simulink model "kalman"  (R2020b)
settings: Solver=VariableStepAuto  StartTime=0.0  StopTime=60  RelTol=1e-3
values from neighbouring files (symbols this model uses):
  dt_sample = 0.01    [main.m]
  dt_sensor = 5    [main.m]
  dt_sim = 0.001    [main.m]
  J = 0.7    [main.m]
  P0 = diag([(10*pi/180)^2;(1*pi/180)^2])    [main.m]
  seedv = randi(2^32)    [main.m]
  seedw = randi(2^32)    [main.m]
  sigmav = 1*pi/180    (= 0.0174532925199)    [main.m]
  sigmaw = 0.001    [main.m]
  x0_hat = [0;0]    [main.m]
libraries: simulink x1
settings Model: Creator=tjones  LastModifiedBy=tjones

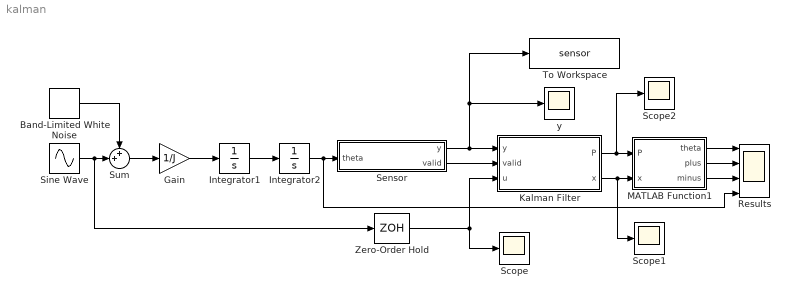
== system kalman ==
  Band-Limited White Noise : simulink/Sources/Band-Limited White Noise  Cov=[sigmaw^2]  Ts=dt_sim  seed=[seedw]
  Gain : Gain  Gain=1/J
  Integrator1 : Integrator
  Integrator2 : Integrator
  Kalman Filter : Subsystem
  MATLAB Function1 : MATLAB Function  TreatAsAtomicUnit=on
  Results : Scope  NumInputPorts=4
  Scope : Scope
  Scope1 : Scope
  Scope2 : Scope
  Sensor : Subsystem
  Sine Wave : Sin  Amplitude=0  SampleTime=dt_sim
  Sum : Sum  Inputs=++|
  To Workspace : ToWorkspace  VariableName=sensor  SaveFormat=Timeseries  SampleTime=-1
  Zero-Order Hold : ZeroOrderHold  SampleTime=dt_sample
  y : Scope
  wires:
  Integrator1/1 -> Integrator2/1
  Integrator2/1 -> Results/4, Sensor/1(theta)
  Sensor/1(y) -> Kalman Filter/1(y), y/1, To Workspace/1
  Gain/1 -> Integrator1/1
  Sine Wave/1 -> Sum/2, Zero-Order Hold/1
  Sum/1 -> Gain/1
  Zero-Order Hold/1 -> Scope/1, Kalman Filter/3(u)
  Sensor/2(valid) -> Kalman Filter/2(valid)
  Kalman Filter/1(P) -> Scope2/1, MATLAB Function1/1(P)
  Kalman Filter/2(x) -> Scope1/1, MATLAB Function1/2(x)
  MATLAB Function1/1(theta) -> Results/1
  MATLAB Function1/2(plus) -> Results/2
  MATLAB Function1/3(minus) -> Results/3
  Band-Limited White Noise/1 -> Sum/1

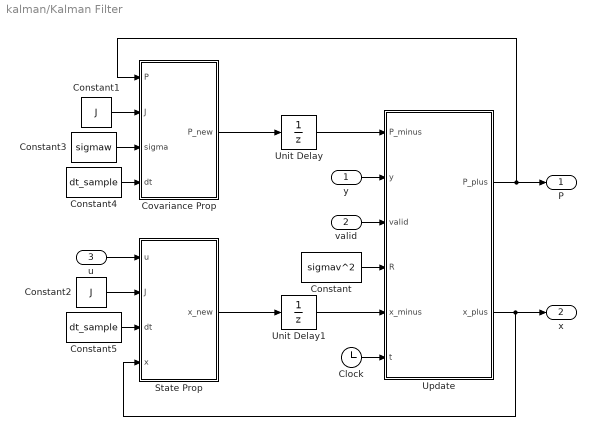
== system kalman/Kalman Filter ==
  y : Inport
  valid : Inport  Port=2
  u : Inport  Port=3
  Clock : Clock
  Constant : Constant  Value=sigmav^2  SampleTime=dt_sample
  Constant1 : Constant  Value=J  SampleTime=dt_sample
  Constant2 : Constant  Value=J  SampleTime=dt_sample
  Constant3 : Constant  Value=sigmaw  SampleTime=dt_sample
  Constant4 : Constant  Value=dt_sample  SampleTime=dt_sample
  Constant5 : Constant  Value=dt_sample  SampleTime=dt_sample
  Covariance Prop : MATLAB Function  TreatAsAtomicUnit=on
  State Prop : MATLAB Function  TreatAsAtomicUnit=on
  Unit Delay : UnitDelay  InitialCondition=P0  SampleTime=dt_sample  HasFrameUpgradeWarning=on
  Unit Delay1 : UnitDelay  InitialCondition=x0_hat  SampleTime=dt_sample  HasFrameUpgradeWarning=on
  Update : MATLAB Function  TreatAsAtomicUnit=on
  P : Outport
  x : Outport  Port=2
  wires:
  Covariance Prop/1(P_new) -> Unit Delay/1
  State Prop/1(x_new) -> Unit Delay1/1
  Constant/1 -> Update/4(R)
  Unit Delay1/1 -> Update/5(x_minus)
  valid/1 -> Update/3(valid)
  u/1 -> State Prop/1(u)
  Constant1/1 -> Covariance Prop/2(J)
  y/1 -> Update/2(y)
  Constant2/1 -> State Prop/2(J)
  Update/2(x_plus) -> x/1, State Prop/4(x)
  Update/1(P_plus) -> Covariance Prop/1(P), P/1
  Unit Delay/1 -> Update/1(P_minus)
  Constant3/1 -> Covariance Prop/3(sigma)
  Clock/1 -> Update/6(t)
  Constant4/1 -> Covariance Prop/4(dt)
  Constant5/1 -> State Prop/3(dt)

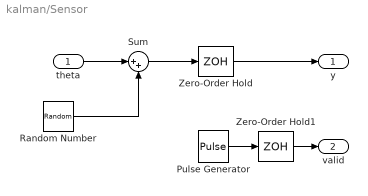
== system kalman/Sensor ==
  theta : Inport
  Pulse Generator : DiscretePulseGenerator  PulseType=Time based  Period=dt_sensor  PulseWidth=dt_sample/dt_sensor*100
  Random Number : RandomNumber  Variance=sigmav^2  Seed=seedv  SampleTime=dt_sim
  Sum : Sum  Inputs=|++
  Zero-Order Hold : ZeroOrderHold  SampleTime=dt_sample
  Zero-Order Hold1 : ZeroOrderHold  SampleTime=dt_sample
  y : Outport
  valid : Outport  Port=2
  wires:
  theta/1 -> Sum/1
  Random Number/1 -> Sum/2
  Sum/1 -> Zero-Order Hold/1
  Zero-Order Hold/1 -> y/1
  Pulse Generator/1 -> Zero-Order Hold1/1
  Zero-Order Hold1/1 -> valid/1

== matlab function kalman/Kalman Filter/Covariance Prop ==
  data: P input; P_new output; J input; sigma input; dt input
function P_new = fcn(P,J,sigma,dt)

Phi = [1, dt; 0, 1];

sig2 = sigma^2;
J2 = J^2;
Qd = [(sig2*dt^3)/(3*J2), (sig2*dt^2)/(2*J2);
      (sig2*dt^2)/(2*J2), (sig2*dt)/J2];

P_new = Phi*P*Phi' + Qd;

== matlab function kalman/Kalman Filter/State Prop ==
  data: u input; x_new output; J input; dt input; x input
function x_new = fcn(u, J, dt, x)

Phi = [1, dt; 0, 1];

Bd = [dt^2/(2*J); dt/J];

x_new = Phi*x + Bd*u;

== matlab function kalman/Kalman Filter/Update ==
  data: P_minus input; P_plus output; y input; valid input; R input; x_minus input; t input; x_plus output
function [P_plus, x_plus] = fcn(P_minus,y,valid,R,x_minus,t)

if valid == 1 && t ~= 0

    H = [1,0];

%     P_temp = [P_minus(1,1), P_minus(1,2);
%               P_minus(2,1), P_minus(2,2)];
%     K0 = P_temp*H';
%     K1 = H*P_minus*H' + R;
%     K = K0/K1;

    K = (P_minus*H')/(H*P_minus*H' + R); % Equation E.126

    x_plus = x_minus + K*(y-H*x_minus); % x[k]=x[k-1]+K*residual (Eq E.122)

    P_plus = (eye(2) - K*H)*P_minus; % Equation E.127

else % no new sensor reading

    % act as a pass through
    P_plus = P_minus;
    x_plus = x_minus;
end

== matlab function kalman/MATLAB Function1 ==
  data: P input; theta output; x input; plus output; minus output
function [theta, plus, minus] = fcn(P, x)

theta = x(1);
plus = theta + 3*sqrt(P(1,1));
minus = theta - 3*sqrt(P(1,1));
